simulink model "ServoMotor_Updated_version"  (R2024a)
settings: Solver=ode15s  StartTime=0.0  StopTime=10.0  RelTol=1e-3
model workspace (MAT data in the model file):
  J = 5e-05
  L = 0.01
  R = 4
  b = 0.0005
  k = 0.2
  ki = 7.33
  kp = 9.39
  ts = 0.1
  v = 7.4
libraries: SignalEditorBlockLib x1
settings Model: Creator=awabm  LastModifiedBy=awabm

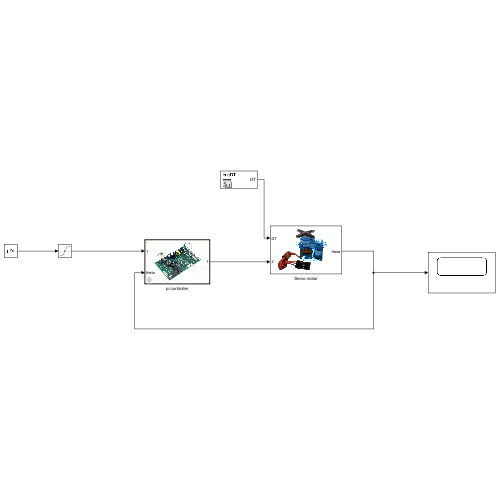
[thumbnail: Simulink's stored preview of the top-level diagram]
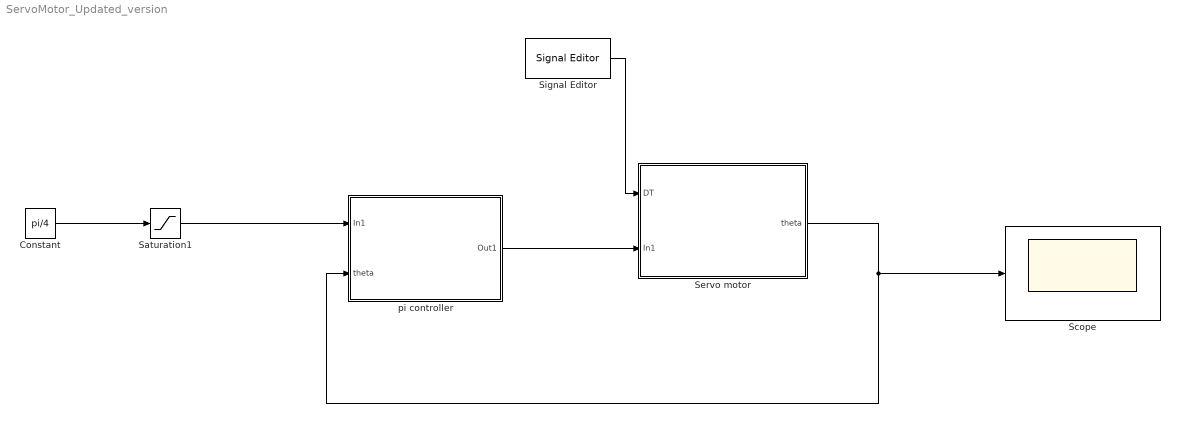
== system ServoMotor_Updated_version ==
  Constant : Constant  Value=pi/4
  Saturation1 : Saturate  UpperLimit=pi/4  LowerLimit=-pi/4
  Scope : Scope
  Servo motor : Subsystem
      mask Display: image('Micro_servo.jpg');
  Signal Editor : SignalEditorBlockLib/Signal Editor  FileName=C:\Users\awabm\OneDrive\سطح المكتب\Coursera\Modeling and Simulation with Simulink\Creating Test Scenarios and Comparing Simulations_2\DT.mat  ActiveScenario=largDT  ActiveSignal=DT  IsBus=off  OutputBusObjectStr=Bus: BusObject  SampleTime=0  Interpolate=off  ZeroCross=off  OutputAfterFinalValue=Setting to zero  Unit=inherit  PreserveSignalName=on  ApplySigPropsToAllScenarios=on  ApplySigPropsToAllSignals=off
  pi controller : Subsystem  TreatAsAtomicUnit=on  mask{kp=9.39, ki=7.33, ts=.01}
      mask prompts: kp "proportional gain"; ki "integral gain"; ts "sample time"
      mask Display: image('1575270966_s-l1600.jpg');
  wires:
  Constant/1 -> Saturation1/1
  Servo motor/1(theta) -> pi controller/2(theta), Scope/1
  Saturation1/1 -> pi controller/1(In1)
  pi controller/1(Out1) -> Servo motor/2(In1)
  Signal Editor/1 -> Servo motor/1(DT)

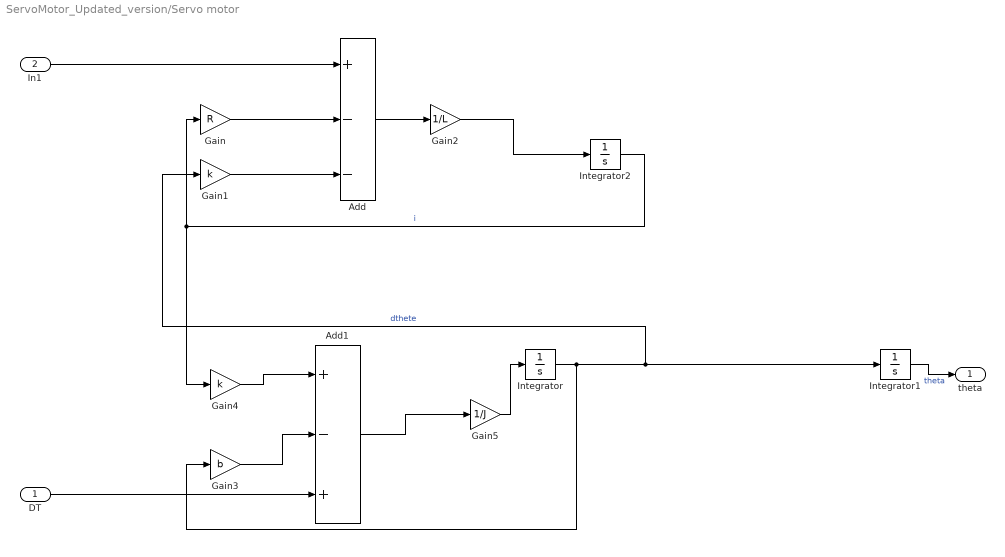
== system ServoMotor_Updated_version/Servo motor ==
  DT : Inport
  In1 : Inport  Port=2
  Add : Sum  Inputs=+--
  Add1 : Sum  Inputs=+-+
  Gain : Gain  Gain=R
  Gain1 : Gain  Gain=k
  Gain2 : Gain  Gain=1/L
  Gain3 : Gain  Gain=b
  Gain4 : Gain  Gain=k
  Gain5 : Gain  Gain=1/J
  Integrator : Integrator
  Integrator1 : Integrator
  Integrator2 : Integrator
  theta : Outport
  wires:
  Integrator/1 -> Gain3/1, Integrator1/1, Gain1/1  "dthete"
  Integrator2/1 -> Gain4/1, Gain/1  "i"
  Gain5/1 -> Integrator/1
  Gain3/1 -> Add1/2
  Add1/1 -> Gain5/1
  Gain/1 -> Add/2
  Add/1 -> Gain2/1
  Gain4/1 -> Add1/1
  In1/1 -> Add/1
  Gain1/1 -> Add/3
  Gain2/1 -> Integrator2/1
  Integrator1/1 -> theta/1  "theta"
  DT/1 -> Add1/3

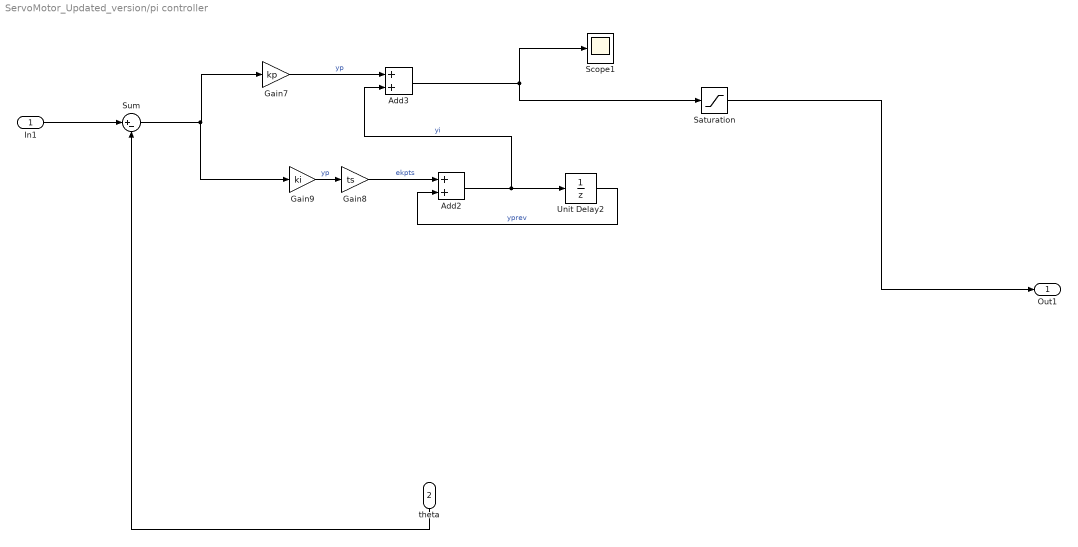
== system ServoMotor_Updated_version/pi controller ==
  In1 : Inport
  theta : Inport  Port=2
  Add2 : Sum
  Add3 : Sum
  Gain7 : Gain  Gain=kp
  Gain8 : Gain  Gain=ts
  Gain9 : Gain  Gain=ki
  Saturation : Saturate  UpperLimit=v  LowerLimit=-v
  Scope1 : Scope
  Sum : Sum  Inputs=|+-
  Unit Delay2 : UnitDelay  SampleTime=ts  HasFrameUpgradeWarning=on
  Out1 : Outport
  wires:
  Add2/1 -> Add3/2, Unit Delay2/1  "yi"
  Unit Delay2/1 -> Add2/2  "yprev"
  Gain7/1 -> Add3/1  "yp"
  Gain8/1 -> Add2/1  "ekpts"
  Sum/1 -> Gain9/1, Gain7/1
  Add3/1 -> Saturation/1, Scope1/1
  Saturation/1 -> Out1/1
  Gain9/1 -> Gain8/1  "yp"
  theta/1 -> Sum/2
  In1/1 -> Sum/1
